simulink model "DistanceCalculation_Module"  (R2026a)
settings: Solver=VariableStepAuto  StopTime=30
undefined symbols (not defined in the file): D_noLead_m
libraries: simulink x1
settings Model: Creator=ADMIN  LastModifiedBy=ASUS

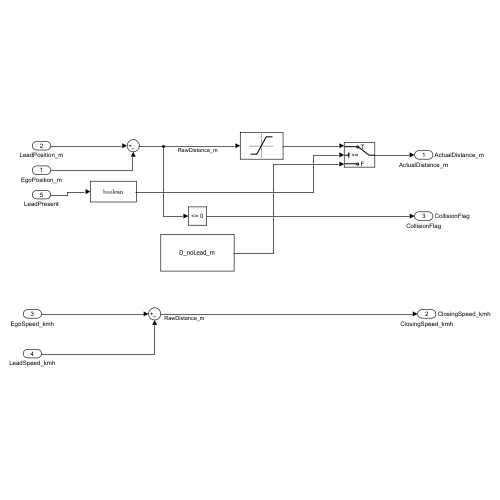
[thumbnail: Simulink's stored preview of the top-level diagram]
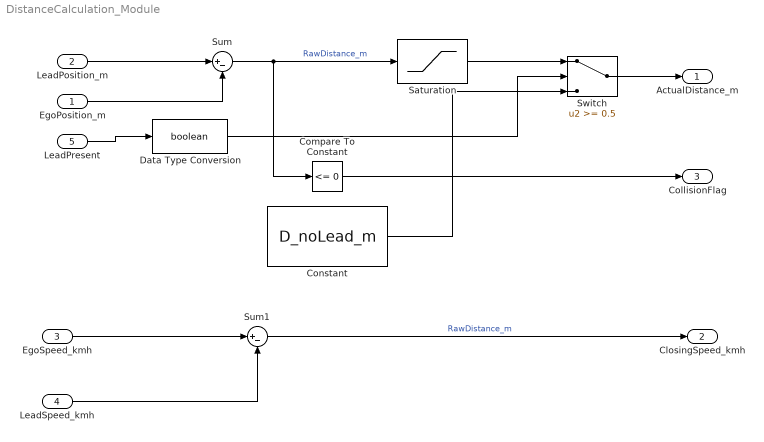
== system DistanceCalculation_Module ==
  EgoPosition_m : Inport
  LeadPosition_m : Inport  Port=2
  EgoSpeed_kmh : Inport  Port=3
  LeadSpeed_kmh : Inport  Port=4
  LeadPresent : Inport  Port=5
  Compare To Constant : simulink/Logic and Bit Operations/Compare To Constant  relop=<=  const=0  OutDataTypeStr=boolean
  Constant : Constant  Value=D_noLead_m
  Data Type Conversion : DataTypeConversion  OutDataTypeStr=boolean  SaturateOnIntegerOverflow=off  RndMeth=Floor
  Saturation : Saturate  UpperLimit=inf  LowerLimit=0
  Sum : Sum  Inputs=|+-
  Sum1 : Sum  Inputs=|+-
  Switch : Switch  Threshold=0.5  SaturateOnIntegerOverflow=off  InputSameDT=off
  ActualDistance_m : Outport  SignalName=ActualDistance_m
  ClosingSpeed_kmh : Outport  Port=2  SignalName=ClosingSpeed_kmh
  CollisionFlag : Outport  Port=3  SignalName=CollisionFlag
  wires:
  LeadPosition_m/1 -> Sum/1
  EgoPosition_m/1 -> Sum/2
  Sum/1 -> Saturation/1, Compare To Constant/1  "RawDistance_m"
  EgoSpeed_kmh/1 -> Sum1/1
  LeadSpeed_kmh/1 -> Sum1/2
  Saturation/1 -> Switch/1
  Constant/1 -> Switch/3
  Sum1/1 -> ClosingSpeed_kmh/1  "RawDistance_m"
  Switch/1 -> ActualDistance_m/1
  Compare To Constant/1 -> CollisionFlag/1
  LeadPresent/1 -> Data Type Conversion/1
  Data Type Conversion/1 -> Switch/2
